simulink model "quadcopter"  (R2022b)
settings: Solver=VariableStepAuto  StartTime=0  StopTime=5  FixedStep=0.00000001  RelTol=1e-3  EnableMultiTasking=on
libraries: slpidlib x4, aerolibutil x2, shared6dof x1, aerolibanimutils x1, vrlib x1
settings Model: Creator=The MathWorks, Inc.  LastModifiedBy=aadri
settings SolverCC: AlgebraicLoopSolver=TrustRegion
settings DataIOCC: LimitDataPoints=on  SaveFormat=Array  SaveOutput=off  SignalLogging=off  DSMLogging=off  SaveTime=off  ReturnWorkspaceOutputs=off
settings OptimizationCC: BlockReduction=off  BufferReuse=off  LifeSpan=inf
settings DebuggingCC: AlgebraicLoopMsg=none  ParameterPrecisionLossMsg=none  AllowSymbolicDim=off  PregeneratedLibrarySubsystemCodeDiagnostic=none  SFUnexpectedBacktrackingDiag=warning  SFNoUnconditionalDefaultTransitionDiag=warning  SFExecutionAtInitializationDiag=none  SFMachineParentedDataDiag=warning  ArithmeticOperatorsInVariantConditions=warning
settings HardwareCC: ProdBitPerPointer=32  ProdBitPerSizeT=32  ProdBitPerPtrDiffT=32  ProdLargestAtomicFloat=None  ProdIntDivRoundTo=Undefined  ProdEndianess=Unspecified  ProdWordSize=32  ProdHWDeviceType=32-bit Generic
settings ModelReferenceCC: EnableRefExpFcnMdlSchedulingChecks=on  PropagateSignalLabelsOutOfModel=off
settings SFSimCC: SimUseLocalCustomCode=off  CustomCodeUndefinedFunction=UseInterfaceOnly
settings RTWCC: RTWUseLocalCustomCode=off  DLArmComputeVersion=19.05
settings CodeAppCC: StateflowObjectComments=on
settings GRTTargetCC: TargetLangStandard=C89/C90 (ANSI)
settings ConfigComp: CovMetricSettings=dw  CovSaveCumulativeToWorkspaceVar=on  CovSaveSingleToWorkspaceVar=on  CovExternalEMLEnable=off  CovSFcnEnable=off

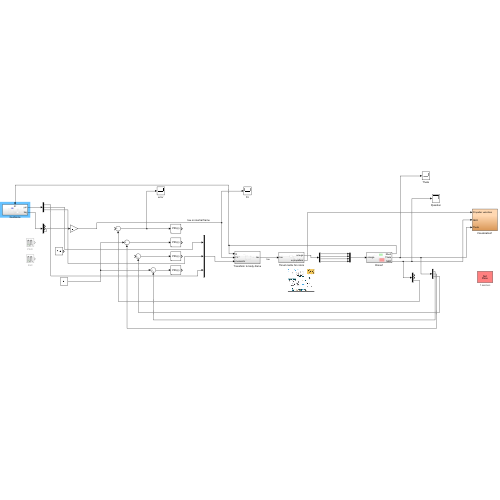
[thumbnail: Simulink's stored preview of the top-level diagram]
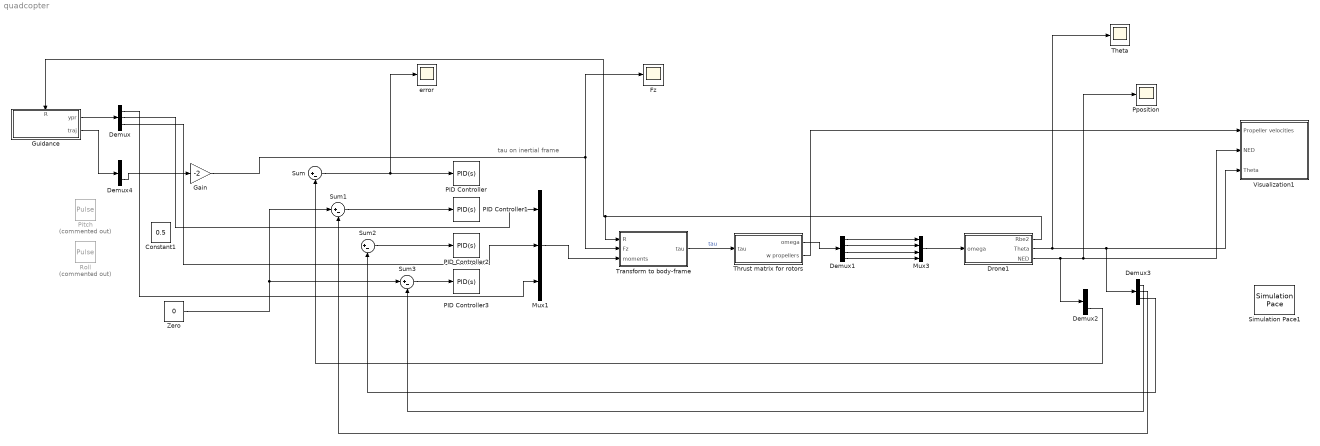
== system quadcopter ==
  note: tau on inertial frame
  Constant1 : Constant  Value=0.5
  Demux{,2..4} (4 alike) : Demux  Outputs=3
  Demux1 : Demux
  Drone1 : Subsystem
  Fz : Scope
  Gain : Gain  Gain=-2
  Guidance : Subsystem
      settings: PortSchema="{\"entries\":[{\"content\":{\"sides\":[{\"content\":{\"connectorIds\":[]},\"type\":\"ConnectorPlacement.EquallySpacedRectSide\",\"uuid\":\"71e90d44-93d9-4948-9515-e584c9c45b4d\"},{\"content\":{\"connectorIds\":[\"Out1\",\"Out2\"],\"side\":\"RIGHT\"},\"type\":\"ConnectorPlacement.EquallySpacedRectSide\",\"uuid\":\"b9ea6ff8-0025-4fb1-8de2-d026a39c77e0\"},{\"content\":{\"connectorIds\":[\"In1\"],\"side\":\"TOP\"},\"type\":\"ConnectorPlacement.EquallySpacedRectSide\",\"uuid\":\"2df58e0f-8a84-452f-95a8-5600226ef525\"}]},\"type\":\"ConnectorPlacement.EquallySpacedConnector\",\"uuid\":\"56107e1d-4b44-4050-8dfa-9220952eccff\"}],\"packageUris\":[\"http://schema.mathworks.com/mf0/Connector/R2020b\"],\"version\":\"1.0\"}"
  Mux1 : Mux  Inputs=3
  Mux3 : Mux
  PID Controller : slpidlib/PID Controller  Controller=PID  Form=Parallel  TimeDomain=Continuous-time  UseExternalTs=off  SampleTime=-1  IntegratorMethod=Forward Euler  FilterMethod=Forward Euler  ControllerParametersSource=internal  P=2  I=0  UseKiTs=off  D=0.5  N=100  UseFilter=on  TunerSelectOption=Transfer Function Based (PID Tuner App)  InitialConditionSource=internal  InitialConditionForIntegrator=0  InitialConditionForFilter=0  DifferentiatorICPrevScaledInput=0  ExternalReset=none  TrackingMode=off  Kt=1  LimitOutput=off  SatLimitsSource=internal  UpperSaturationLimit=5  LowerSaturationLimit=-5  LinearizeAsGain=on  AntiWindupMode=none  Kb=1  LimitIntegrator=off  UpperIntegratorSaturationLimit=inf  LowerIntegratorSaturationLimit=-inf  POutMin=[]  POutMax=[]  IOutMin=[]  IOutMax=[]  DOutMin=[]  DOutMax=[]  NOutMin=[]  NOutMax=[]  SumOutMin=[]  SumOutMax=[]  SaturationOutMin=[]  SaturationOutMax=[]  PParamMin=[]  PParamMax=[]  IParamMin=[]  IParamMax=[]  DParamMin=[]  DParamMax=[]  NParamMin=[]  NParamMax=[]  KbParamMin=[]  KbParamMax=[]  KtParamMin=[]  KtParamMax=[]  KbOutMin=[]  KbOutMax=[]  KtOutMin=[]  KtOutMax=[]  IntegratorOutMin=[]  IntegratorOutMax=[]  FilterOutMin=[]  FilterOutMax=[]  SumI1OutMin=[]  SumI1OutMax=[]  SumI2OutMin=[]  SumI2OutMax=[]  SumI3OutMin=[]  SumI3OutMax=[]  SumI4OutMin=[]  SumI4OutMax=[]  SumDOutMin=[]  SumDOutMax=[]  DifferentiatorOutMin=[]  DifferentiatorOutMax=[]  FilterDiffOutCoefMin=[]  FilterDiffOutCoefMax=[]  ReciprocalOutMin=[]  ReciprocalOutMax=[]  SumDenOutMin=[]  SumDenOutMax=[]  SumNumOutMin=[]  SumNumOutMax=[]  DivideOutMin=[]  DivideOutMax=[]  UdiffTsProdOutMin=[]  UdiffTsProdOutMax=[]  NTsProdOutMin=[]  NTsProdOutMax=[]  UintegralTsProdOutMin=[]  UintegralTsProdOutMax=[]  UngainTsProdOutMin=[]  UngainTsProdOutMax=[]  ClampingZeroOutDataTypeStr=Inherit: Inherit via back propagation  ClampingZeroOutMin=[]  ClampingZeroOutMax=[]  FilterDenConstantOutDataTypeStr=Inherit: Inherit via back propagation  FilterDenConstantOutMin=[]  FilterDenConstantOutMax=[]  PCopyOutDataTypeStr=Inherit: Inherit via back propagation  PCopyOutMin=[]  PCopyOutMax=[]  NCopyOutDataTypeStr=Inherit: Inherit via back propagation  NCopyOutMin=[]  NCopyOutMax=[]  IntegratorContinuousStateAttributes=''  IntegratorStateMustResolveToSignalObject=off  IntegratorRTWStateStorageClass=Auto  FilterContinuousStateAttributes=''  FilterStateMustResolveToSignalObject=off  FilterRTWStateStorageClass=Auto  ParallelPVariant=InternalParameters  IdealPVariant=Disabled  IVariant=InternalParameters  DVariant=InternalParameters  IntegratorVariant=Continuous  SatVariant=Disabled  AWVariant=Passthrough  PCopyVariant=Disabled  TRVariant=Disabled  FdbkBlocksVariant=Forward  IdealPFdbkVariant=Disabled  SatFdbkVariant=Disabled  DerivativeFilterVariant=ContFilter  NVariant=InternalParameters  NCopyVariant=Disabled  FilterICVariant=InternalICsFilter  IntegratorICVariant=InternalICs  ExternalResetVariant=Disabled  TRSumVariant=Passthrough  SumFdbkVariant=Disabled  SumVariant=Sum_PID  TsampFilterVariant=InternalTs  TsampNgainVariant=Passthrough  TsampIntegralVariant=Passthrough  ExternalSaturationOutDataTypeStr=Inherit: Same as second input
  PID Controller1 : slpidlib/PID Controller  Controller=PID  Form=Parallel  TimeDomain=Continuous-time  UseExternalTs=off  SampleTime=-1  IntegratorMethod=Forward Euler  FilterMethod=Forward Euler  ControllerParametersSource=internal  P=2  I=0  UseKiTs=off  D=0.5  N=100  UseFilter=on  TunerSelectOption=Transfer Function Based (PID Tuner App)  InitialConditionSource=internal  InitialConditionForIntegrator=0  InitialConditionForFilter=0  DifferentiatorICPrevScaledInput=0  ExternalReset=none  TrackingMode=off  Kt=1  LimitOutput=off  SatLimitsSource=internal  UpperSaturationLimit=inf  LowerSaturationLimit=-inf  LinearizeAsGain=on  AntiWindupMode=none  Kb=1  LimitIntegrator=off  UpperIntegratorSaturationLimit=inf  LowerIntegratorSaturationLimit=-inf  POutMin=[]  POutMax=[]  IOutMin=[]  IOutMax=[]  DOutMin=[]  DOutMax=[]  NOutMin=[]  NOutMax=[]  SumOutMin=[]  SumOutMax=[]  SaturationOutMin=[]  SaturationOutMax=[]  PParamMin=[]  PParamMax=[]  IParamMin=[]  IParamMax=[]  DParamMin=[]  DParamMax=[]  NParamMin=[]  NParamMax=[]  KbParamMin=[]  KbParamMax=[]  KtParamMin=[]  KtParamMax=[]  KbOutMin=[]  KbOutMax=[]  KtOutMin=[]  KtOutMax=[]  IntegratorOutMin=[]  IntegratorOutMax=[]  FilterOutMin=[]  FilterOutMax=[]  SumI1OutMin=[]  SumI1OutMax=[]  SumI2OutMin=[]  SumI2OutMax=[]  SumI3OutMin=[]  SumI3OutMax=[]  SumI4OutMin=[]  SumI4OutMax=[]  SumDOutMin=[]  SumDOutMax=[]  DifferentiatorOutMin=[]  DifferentiatorOutMax=[]  FilterDiffOutCoefMin=[]  FilterDiffOutCoefMax=[]  ReciprocalOutMin=[]  ReciprocalOutMax=[]  SumDenOutMin=[]  SumDenOutMax=[]  SumNumOutMin=[]  SumNumOutMax=[]  DivideOutMin=[]  DivideOutMax=[]  UdiffTsProdOutMin=[]  UdiffTsProdOutMax=[]  NTsProdOutMin=[]  NTsProdOutMax=[]  UintegralTsProdOutMin=[]  UintegralTsProdOutMax=[]  UngainTsProdOutMin=[]  UngainTsProdOutMax=[]  ClampingZeroOutDataTypeStr=Inherit: Inherit via back propagation  ClampingZeroOutMin=[]  ClampingZeroOutMax=[]  FilterDenConstantOutDataTypeStr=Inherit: Inherit via back propagation  FilterDenConstantOutMin=[]  FilterDenConstantOutMax=[]  PCopyOutDataTypeStr=Inherit: Inherit via back propagation  PCopyOutMin=[]  PCopyOutMax=[]  NCopyOutDataTypeStr=Inherit: Inherit via back propagation  NCopyOutMin=[]  NCopyOutMax=[]  IntegratorContinuousStateAttributes=''  IntegratorStateMustResolveToSignalObject=off  IntegratorRTWStateStorageClass=Auto  FilterContinuousStateAttributes=''  FilterStateMustResolveToSignalObject=off  FilterRTWStateStorageClass=Auto  ParallelPVariant=InternalParameters  IdealPVariant=Disabled  IVariant=InternalParameters  DVariant=InternalParameters  IntegratorVariant=Continuous  SatVariant=Disabled  AWVariant=Passthrough  PCopyVariant=Disabled  TRVariant=Disabled  FdbkBlocksVariant=Forward  IdealPFdbkVariant=Disabled  SatFdbkVariant=Disabled  DerivativeFilterVariant=ContFilter  NVariant=InternalParameters  NCopyVariant=Disabled  FilterICVariant=InternalICsFilter  IntegratorICVariant=InternalICs  ExternalResetVariant=Disabled  TRSumVariant=Passthrough  SumFdbkVariant=Disabled  SumVariant=Sum_PID  TsampFilterVariant=InternalTs  TsampNgainVariant=Passthrough  TsampIntegralVariant=Passthrough  ExternalSaturationOutDataTypeStr=Inherit: Same as second input
  PID Controller2 : slpidlib/PID Controller  Controller=PID  Form=Parallel  TimeDomain=Continuous-time  UseExternalTs=off  SampleTime=-1  IntegratorMethod=Forward Euler  FilterMethod=Forward Euler  ControllerParametersSource=internal  P=4  I=0  UseKiTs=off  D=2  N=100  UseFilter=on  TunerSelectOption=Transfer Function Based (PID Tuner App)  InitialConditionSource=internal  InitialConditionForIntegrator=0  InitialConditionForFilter=0  DifferentiatorICPrevScaledInput=0  ExternalReset=none  TrackingMode=off  Kt=1  LimitOutput=off  SatLimitsSource=internal  UpperSaturationLimit=inf  LowerSaturationLimit=-inf  LinearizeAsGain=on  AntiWindupMode=none  Kb=1  LimitIntegrator=off  UpperIntegratorSaturationLimit=inf  LowerIntegratorSaturationLimit=-inf  POutMin=[]  POutMax=[]  IOutMin=[]  IOutMax=[]  DOutMin=[]  DOutMax=[]  NOutMin=[]  NOutMax=[]  SumOutMin=[]  SumOutMax=[]  SaturationOutMin=[]  SaturationOutMax=[]  PParamMin=[]  PParamMax=[]  IParamMin=[]  IParamMax=[]  DParamMin=[]  DParamMax=[]  NParamMin=[]  NParamMax=[]  KbParamMin=[]  KbParamMax=[]  KtParamMin=[]  KtParamMax=[]  KbOutMin=[]  KbOutMax=[]  KtOutMin=[]  KtOutMax=[]  IntegratorOutMin=[]  IntegratorOutMax=[]  FilterOutMin=[]  FilterOutMax=[]  SumI1OutMin=[]  SumI1OutMax=[]  SumI2OutMin=[]  SumI2OutMax=[]  SumI3OutMin=[]  SumI3OutMax=[]  SumI4OutMin=[]  SumI4OutMax=[]  SumDOutMin=[]  SumDOutMax=[]  DifferentiatorOutMin=[]  DifferentiatorOutMax=[]  FilterDiffOutCoefMin=[]  FilterDiffOutCoefMax=[]  ReciprocalOutMin=[]  ReciprocalOutMax=[]  SumDenOutMin=[]  SumDenOutMax=[]  SumNumOutMin=[]  SumNumOutMax=[]  DivideOutMin=[]  DivideOutMax=[]  UdiffTsProdOutMin=[]  UdiffTsProdOutMax=[]  NTsProdOutMin=[]  NTsProdOutMax=[]  UintegralTsProdOutMin=[]  UintegralTsProdOutMax=[]  UngainTsProdOutMin=[]  UngainTsProdOutMax=[]  ClampingZeroOutDataTypeStr=Inherit: Inherit via back propagation  ClampingZeroOutMin=[]  ClampingZeroOutMax=[]  FilterDenConstantOutDataTypeStr=Inherit: Inherit via back propagation  FilterDenConstantOutMin=[]  FilterDenConstantOutMax=[]  PCopyOutDataTypeStr=Inherit: Inherit via back propagation  PCopyOutMin=[]  PCopyOutMax=[]  NCopyOutDataTypeStr=Inherit: Inherit via back propagation  NCopyOutMin=[]  NCopyOutMax=[]  IntegratorContinuousStateAttributes=''  IntegratorStateMustResolveToSignalObject=off  IntegratorRTWStateStorageClass=Auto  FilterContinuousStateAttributes=''  FilterStateMustResolveToSignalObject=off  FilterRTWStateStorageClass=Auto  ParallelPVariant=InternalParameters  IdealPVariant=Disabled  IVariant=InternalParameters  DVariant=InternalParameters  IntegratorVariant=Continuous  SatVariant=Disabled  AWVariant=Passthrough  PCopyVariant=Disabled  TRVariant=Disabled  FdbkBlocksVariant=Forward  IdealPFdbkVariant=Disabled  SatFdbkVariant=Disabled  DerivativeFilterVariant=ContFilter  NVariant=InternalParameters  NCopyVariant=Disabled  FilterICVariant=InternalICsFilter  IntegratorICVariant=InternalICs  ExternalResetVariant=Disabled  TRSumVariant=Passthrough  SumFdbkVariant=Disabled  SumVariant=Sum_PID  TsampFilterVariant=InternalTs  TsampNgainVariant=Passthrough  TsampIntegralVariant=Passthrough  ExternalSaturationOutDataTypeStr=Inherit: Same as second input
  PID Controller3 : slpidlib/PID Controller  Controller=PID  Form=Parallel  TimeDomain=Continuous-time  UseExternalTs=off  SampleTime=-1  IntegratorMethod=Forward Euler  FilterMethod=Forward Euler  ControllerParametersSource=internal  P=1  I=1  UseKiTs=off  D=0  N=100  UseFilter=on  TunerSelectOption=Transfer Function Based (PID Tuner App)  InitialConditionSource=internal  InitialConditionForIntegrator=0  InitialConditionForFilter=0  DifferentiatorICPrevScaledInput=0  ExternalReset=none  TrackingMode=off  Kt=1  LimitOutput=off  SatLimitsSource=internal  UpperSaturationLimit=inf  LowerSaturationLimit=-inf  LinearizeAsGain=on  AntiWindupMode=none  Kb=1  LimitIntegrator=off  UpperIntegratorSaturationLimit=inf  LowerIntegratorSaturationLimit=-inf  POutMin=[]  POutMax=[]  IOutMin=[]  IOutMax=[]  DOutMin=[]  DOutMax=[]  NOutMin=[]  NOutMax=[]  SumOutMin=[]  SumOutMax=[]  SaturationOutMin=[]  SaturationOutMax=[]  PParamMin=[]  PParamMax=[]  IParamMin=[]  IParamMax=[]  DParamMin=[]  DParamMax=[]  NParamMin=[]  NParamMax=[]  KbParamMin=[]  KbParamMax=[]  KtParamMin=[]  KtParamMax=[]  KbOutMin=[]  KbOutMax=[]  KtOutMin=[]  KtOutMax=[]  IntegratorOutMin=[]  IntegratorOutMax=[]  FilterOutMin=[]  FilterOutMax=[]  SumI1OutMin=[]  SumI1OutMax=[]  SumI2OutMin=[]  SumI2OutMax=[]  SumI3OutMin=[]  SumI3OutMax=[]  SumI4OutMin=[]  SumI4OutMax=[]  SumDOutMin=[]  SumDOutMax=[]  DifferentiatorOutMin=[]  DifferentiatorOutMax=[]  FilterDiffOutCoefMin=[]  FilterDiffOutCoefMax=[]  ReciprocalOutMin=[]  ReciprocalOutMax=[]  SumDenOutMin=[]  SumDenOutMax=[]  SumNumOutMin=[]  SumNumOutMax=[]  DivideOutMin=[]  DivideOutMax=[]  UdiffTsProdOutMin=[]  UdiffTsProdOutMax=[]  NTsProdOutMin=[]  NTsProdOutMax=[]  UintegralTsProdOutMin=[]  UintegralTsProdOutMax=[]  UngainTsProdOutMin=[]  UngainTsProdOutMax=[]  ClampingZeroOutDataTypeStr=Inherit: Inherit via back propagation  ClampingZeroOutMin=[]  ClampingZeroOutMax=[]  FilterDenConstantOutDataTypeStr=Inherit: Inherit via back propagation  FilterDenConstantOutMin=[]  FilterDenConstantOutMax=[]  PCopyOutDataTypeStr=Inherit: Inherit via back propagation  PCopyOutMin=[]  PCopyOutMax=[]  NCopyOutDataTypeStr=Inherit: Inherit via back propagation  NCopyOutMin=[]  NCopyOutMax=[]  IntegratorContinuousStateAttributes=''  IntegratorStateMustResolveToSignalObject=off  IntegratorRTWStateStorageClass=Auto  FilterContinuousStateAttributes=''  FilterStateMustResolveToSignalObject=off  FilterRTWStateStorageClass=Auto  ParallelPVariant=InternalParameters  IdealPVariant=Disabled  IVariant=InternalParameters  DVariant=InternalParameters  IntegratorVariant=Continuous  SatVariant=Disabled  AWVariant=Passthrough  PCopyVariant=Disabled  TRVariant=Disabled  FdbkBlocksVariant=Forward  IdealPFdbkVariant=Disabled  SatFdbkVariant=Disabled  DerivativeFilterVariant=ContFilter  NVariant=InternalParameters  NCopyVariant=Disabled  FilterICVariant=InternalICsFilter  IntegratorICVariant=InternalICs  ExternalResetVariant=Disabled  TRSumVariant=Passthrough  SumFdbkVariant=Disabled  SumVariant=Sum_PID  TsampFilterVariant=InternalTs  TsampNgainVariant=Passthrough  TsampIntegralVariant=Passthrough  ExternalSaturationOutDataTypeStr=Inherit: Same as second input
  Pitch : DiscretePulseGenerator  Commented=on  PulseType=Time based  Amplitude=-0.15  Period=1  PulseWidth=5  PhaseDelay=0.6
  Pposition : Scope
  Roll : DiscretePulseGenerator  Commented=on  PulseType=Time based  Amplitude=0.1  Period=10  PulseWidth=5  PhaseDelay=4
  Simulation Pace1 : aerolibanimutils/Simulation Pace  SimulationPace=1  SleepMode=MATLAB Thread  OutputPaceError=off  SampleTime=0.005
      settings: AttributesFormatString=%<SimulationPace> sec/sec
  Sum{,1..3} (4 alike) : Sum  Inputs=|+-
  Theta : Scope
  Thrust matrix for rotors : Subsystem
  Transform to body-frame : Subsystem
  Visualization1 : Subsystem
  Zero : Constant  Value=0  OutDataTypeStr=Inherit: Inherit via back propagation
  error : Scope
  wires:
  Sum/1 -> error/1, PID Controller/1
  Sum3/1 -> PID Controller3/1
  Drone1/3(NED) -> Demux2/1, Pposition/1, Visualization1/2(NED)
  Demux1/4 -> Mux3/4
  Demux1/3 -> Mux3/3
  Demux1/1 -> Mux3/1
  Mux3/1 -> Drone1/1(omega)
  Transform to body-frame/1(tau) -> Thrust matrix for rotors/1(tau)  "tau"
  Demux1/2 -> Mux3/2
  Sum2/1 -> PID Controller2/1
  Demux2/3 -> Sum/2
  Thrust matrix for rotors/1(omega) -> Demux1/1
  Sum1/1 -> PID Controller1/1
  Drone1/2(Theta) -> Theta/1, Demux3/1, Visualization1/3(Theta)
  Demux3/1 -> Sum3/2
  Demux3/2 -> Sum1/2
  Demux3/3 -> Sum2/2
  Drone1/1(Rbe2) -> Guidance/1(R), Transform to body-frame/1(R)
  Mux1/1 -> Transform to body-frame/3(moments)
  Thrust matrix for rotors/2(w propellers) -> Visualization1/1(Propeller velocities)
  Guidance/1(ypr) -> Demux/1
  Guidance/2(traj) -> Demux4/1
  Demux4/3 -> Gain/1
  Demux/3 -> Mux1/2
  Demux/1 -> Mux1/3
  Demux/2 -> Mux1/1
  Zero/1 -> Sum3/1, Sum1/1
  Gain/1 -> Fz/1, Transform to body-frame/2(Fz)

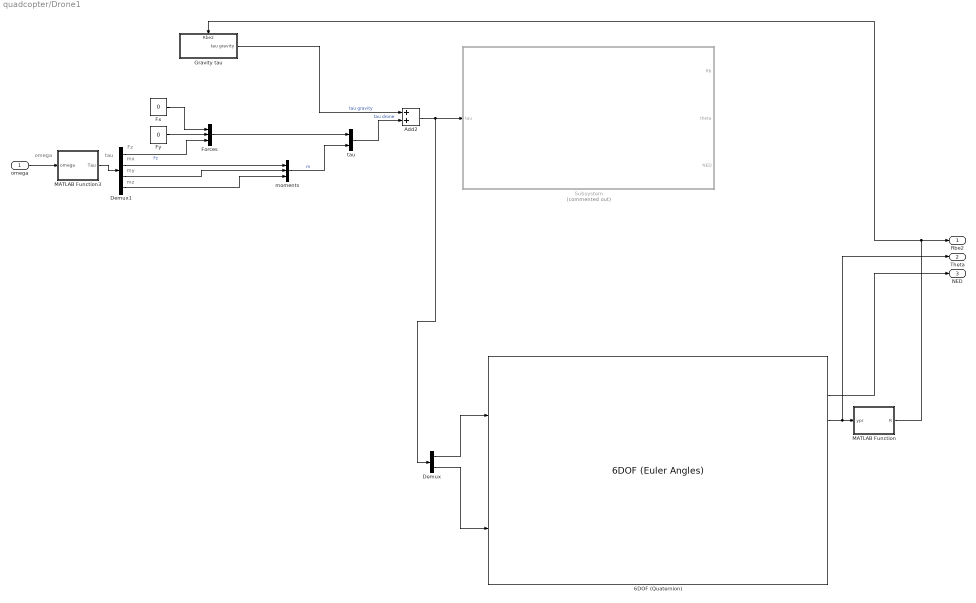
== system quadcopter/Drone1 ==
  note: mx
  note: Fz
  note: omega
  note: tau
  note: my
  note: mz
  omega : Inport
  6DOF (Quaternion) : shared6dof/6DOF (Euler Angles)  units=Metric (MKS)  mtype=Fixed  rep=Euler Angles  xme_0=init.posNED  Vm_0=init.vb  eul_0=init.euler  pm_0=init.angRates  mass_0=Vehicle.Airframe.mass  mass_e=0.5  mass_f=2.0  inertia=Vehicle.Airframe.inertia  inertia_e=eye(3)  inertia_f=2*eye(3)  k_quat=Vehicle.SixDOF.quatGain  vre_flag=on  abi_flag=on  aMode=aMode  xme_statename=''  Vm_statename=''  eul_statename=''  quat_statename=''  pm_statename=''  mass_statename=''
  Add2 : Sum
  Demux : Demux  Outputs=2
  Demux1 : Demux
  Forces : Mux  Inputs=3
  Fx : Constant  Value=0
  Fy : Constant  Value=0
  Gravity tau : Subsystem
      settings: PortSchema="{\"entries\":[{\"content\":{\"sides\":[{\"content\":{\"connectorIds\":[]},\"type\":\"ConnectorPlacement.EquallySpacedRectSide\",\"uuid\":\"34476b71-9b24-4b80-93b9-db525faab568\"},{\"content\":{\"connectorIds\":[\"Out1\"],\"side\":\"RIGHT\"},\"type\":\"ConnectorPlacement.EquallySpacedRectSide\",\"uuid\":\"f9e648e7-9cce-40ff-8639-1a2f2272512c\"},{\"content\":{\"connectorIds\":[\"In1\"],\"side\":\"TOP\"},\"type\":\"ConnectorPlacement.EquallySpacedRectSide\",\"uuid\":\"706437ea-9124-4f20-99e4-286431f5f4e3\"}]},\"type\":\"ConnectorPlacement.EquallySpacedConnector\",\"uuid\":\"20ce1a05-06ad-40f2-848e-d017002622b7\"}],\"packageUris\":[\"http://schema.mathworks.com/mf0/Connector/R2020b\"],\"version\":\"1.0\"}"
  MATLAB Function : MATLAB Function  TreatAsAtomicUnit=on
  MATLAB Function3 : MATLAB Function  TreatAsAtomicUnit=on
  Subsystem : Subsystem  Commented=on
  moments : Mux  Inputs=3
  tau : Mux  Inputs=2
  Rbe2 : Outport
  Theta : Outport  Port=2
  NED : Outport  Port=3
  wires:
  Demux1/2 -> moments/1
  Demux1/3 -> moments/2
  Demux1/4 -> moments/3
  MATLAB Function3/1(Tau) -> Demux1/1
  omega/1 -> MATLAB Function3/1(omega)
  Demux1/1 -> Forces/3  "Fz"
  Fy/1 -> Forces/2
  Fx/1 -> Forces/1
  Forces/1 -> tau/1
  moments/1 -> tau/2  "m"
  Gravity tau/1(tau gravity) -> Add2/1  "tau gravity"
  tau/1 -> Add2/2  "tau drone"
  Add2/1 -> Demux/1, Subsystem/1(tau)
  Demux/1 -> 6DOF (Quaternion)/1
  Demux/2 -> 6DOF (Quaternion)/2
  6DOF (Quaternion)/3 -> Theta/1, MATLAB Function/1(ypr)
  MATLAB Function/1(R) -> Gravity tau/1(Rbe2), Rbe2/1
  6DOF (Quaternion)/2 -> NED/1

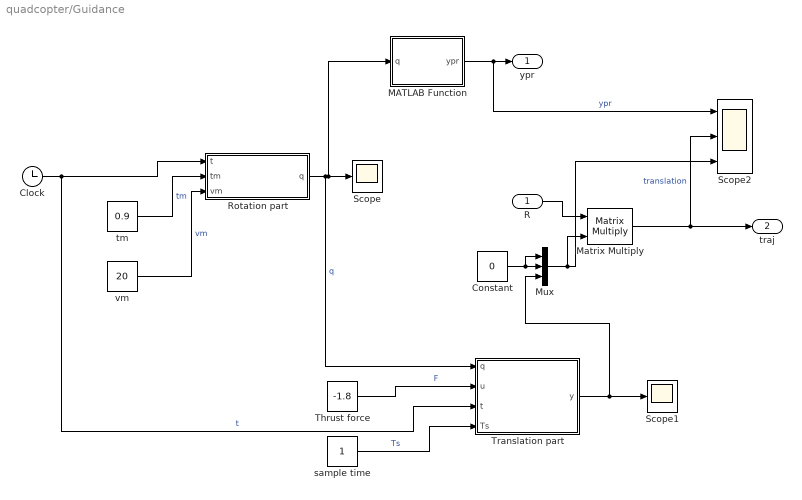
== system quadcopter/Guidance ==
  R : Inport
  Clock : Clock
  Constant : Constant  Value=0
  MATLAB Function : MATLAB Function  TreatAsAtomicUnit=on
  Matrix Multiply : Product  Multiplication=Matrix(*)
  Mux : Mux  Inputs=3
  Rotation part : Subsystem
  Scope : Scope
  Scope1 : Scope
  Scope2 : Scope  NumInputPorts=3
  Thrust force : Constant  Value=-1.8
  Translation part : Subsystem
  sample time : Constant
  tm : Constant  Value=0.9
  vm : Constant  Value=20
  ypr : Outport
  traj : Outport  Port=2
  wires:
  Clock/1 -> Translation part/3(t), Rotation part/1(t)  "t"
  tm/1 -> Rotation part/2(tm)  "tm"
  vm/1 -> Rotation part/3(vm)  "vm"
  Rotation part/1(q) -> Translation part/1(q), MATLAB Function/1(q), Scope/1  "q"
  Thrust force/1 -> Translation part/2(u)  "F"
  sample time/1 -> Translation part/4(Ts)  "Ts"
  Translation part/1(y) -> Mux/3, Scope1/1
  MATLAB Function/1(ypr) -> Scope2/1, ypr/1  "ypr"
  R/1 -> Matrix Multiply/1
  Constant/1 -> Mux/2, Mux/1
  Matrix Multiply/1 -> Scope2/2, traj/1  "translation"
  Mux/1 -> Scope2/3, Matrix Multiply/2

== system quadcopter/Thrust matrix for rotors ==
  note: omega
  note: tau
  tau : Inport
  MATLAB Function : MATLAB Function  TreatAsAtomicUnit=on
  MATLAB Function1 : MATLAB Function  TreatAsAtomicUnit=on
  omega : Outport
  w propellers : Outport  Port=2
  wires:
  tau/1 -> MATLAB Function/1(tau)
  MATLAB Function/1(omega) -> MATLAB Function1/1(omega), omega/1
  MATLAB Function1/1(w) -> w propellers/1

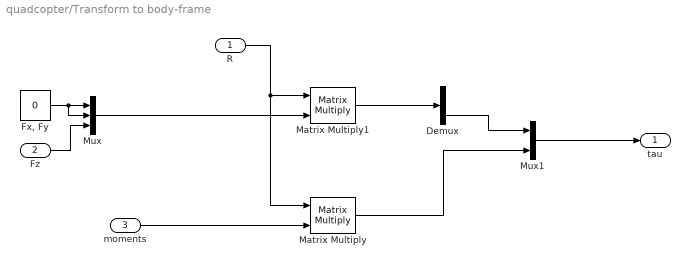
== system quadcopter/Transform to body-frame ==
  R : Inport
  Fz : Inport  Port=2
  moments : Inport  Port=3
  Demux : Demux  Outputs=3
  "Fx, Fy" : Constant  Value=0
  Matrix Multiply : Product  Multiplication=Matrix(*)
  Matrix Multiply1 : Product  Multiplication=Matrix(*)
  Mux : Mux  Inputs=3
  Mux1 : Mux  Inputs=2
  tau : Outport
  wires:
  "Fx, Fy"/1 -> Mux/2, Mux/1
  Fz/1 -> Mux/3
  R/1 -> Matrix Multiply/1, Matrix Multiply1/1
  Mux/1 -> Matrix Multiply1/2
  moments/1 -> Matrix Multiply/2
  Matrix Multiply1/1 -> Demux/1
  Mux1/1 -> tau/1
  Demux/3 -> Mux1/1
  Matrix Multiply/1 -> Mux1/2

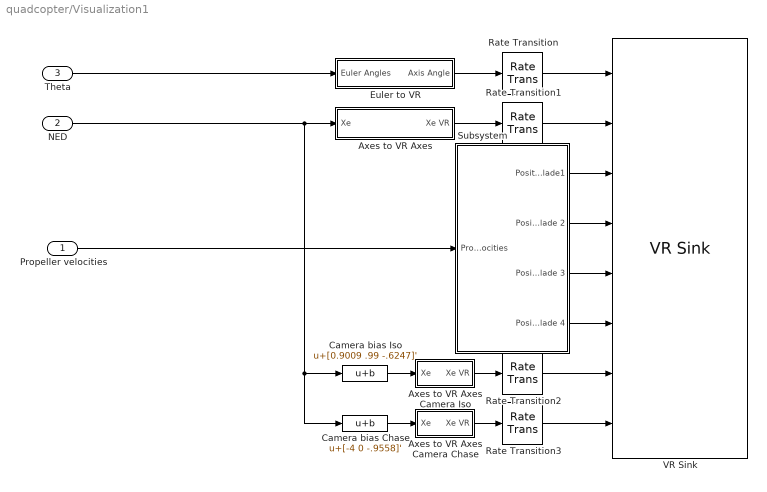
== system quadcopter/Visualization1 ==
  Propeller velocities : Inport
  NED : Inport  Port=2
  Theta : Inport  Port=3
  Axes to VR Axes : Subsystem
  Axes to VR Axes Camera Chase : Subsystem
  Axes to VR Axes Camera Iso : Subsystem
  Camera bias Chase : Bias  Bias=[-4 0 -.9558]'  SaturateOnIntegerOverflow=off
  Camera bias Iso : Bias  Bias=[0.9009 .99 -.6247]'  SaturateOnIntegerOverflow=off
  Euler to VR : Subsystem
  Rate Transition{,1..3} (4 alike) : RateTransition
  Subsystem : Subsystem
  VR Sink : vrlib/VR Sink  InstantiateOnLoad=on  SampleTime=12*0.005  ViewEnable=on  RemoteChange=off  RemoteView=off  FieldsWritten=QuadBody.rotation.4.1.1.double#QuadBody.translation.3.1.1.double#Blade1.rotation.4.1.1.double#Blade3.rotation.4.1.1.double#Blade2.rotation.4.1.1.double#Blade4.rotation.4.1.1.double#IsoNoRotation.position.3.1.1.double#OnQuadNoRotation.position.3.1.1.double  WorldFileName=Quadcopter_VR.wrl  AutoView=on  VideoDimensions=[]  AllowVariableSize=off  FigureProperties="{'Position', 'Name', 'Viewpoint', 'CameraBound', 'CameraDirection', 'CameraPosition', 'CameraUpVector', 'ZoomFactor', 'Antialiasing', 'Headlight', 'Lighting', 'NavPanel', 'Sound', 'StatusBar', 'Stereo3D', 'Stereo3DCameraOffset', 'Stereo3DHIT', 'ToolBar', 'Textures', 'Transparency', 'Triad', 'Wireframe', 'NavZones', 'NavMode', 'NavSpeed', 'CaptureFileFormat', 'CaptureFileName', 'Record2DCompressMethod', 'Record2DCompressQuality', 'Record2D', 'Record2DFileName', 'Record2DFPS'; [1.9871428571428569e+02   4.2642857142857133e+02   5.7600000000000000e+02   3.5000000000000006e+02], '', 'Isometric', 'on', [0.0000000000000000e+00   0.0000000000000000e+00  -1.0000000000000000e+00], [0.0000000000000000e+00   0.0000000000000000e+00   3.0000000000000000e+00], [0.0000000000000000e+00   1.0000000000000000e+00   0.0000000000000000e+00], [1.0000000000000000e+00], 'on', 'on', 'on', 'halfbar', 'on', 'on', 'off', [1.0000000149011612e-01], [0.0000000000000000e+00], 'on', 'on', 'on', 'none', 'off', 'off', 'fly', 'normal', 'tif', '%f_anim_%n.tif', 'auto', [7.5000000000000000e+01], 'off', '%f_anim_%n.avi', 'auto'}"
  wires:
  Propeller velocities/1 -> Subsystem/1(Propeller velocities)
  Euler to VR/1(Axis Angle) -> Rate Transition/1
  Axes to VR Axes/1(Xe VR) -> Rate Transition1/1
  Camera bias Iso/1 -> Axes to VR Axes Camera Iso/1(Xe)
  Camera bias Chase/1 -> Axes to VR Axes Camera Chase/1(Xe)
  Axes to VR Axes Camera Chase/1(Xe VR) -> Rate Transition3/1
  NED/1 -> Camera bias Chase/1, Camera bias Iso/1, Axes to VR Axes/1(Xe)
  Axes to VR Axes Camera Iso/1(Xe VR) -> Rate Transition2/1
  Theta/1 -> Euler to VR/1(Euler Angles)
  Rate Transition/1 -> VR Sink/1
  Rate Transition1/1 -> VR Sink/2
  Subsystem/1(Position Blade1) -> VR Sink/3
  Subsystem/2(Position Blade 2) -> VR Sink/4
  Subsystem/3(Position Blade 3) -> VR Sink/5
  Subsystem/4(Position Blade 4) -> VR Sink/6
  Rate Transition2/1 -> VR Sink/7
  Rate Transition3/1 -> VR Sink/8

== system quadcopter/Drone1/Gravity tau ==
  Rbe2 : Inport
  Constant1 : Constant  Value=[0;0;0.28*9.81]
  Constant2 : Constant  Value=[0;0;0]
  Matrix Multiply : Product  Multiplication=Matrix(*)
  Mux : Mux  Inputs=2
  tau gravity : Outport
  wires:
  Rbe2/1 -> Matrix Multiply/1
  Matrix Multiply/1 -> Mux/1  "tau gravity"
  Mux/1 -> tau gravity/1
  Constant1/1 -> Matrix Multiply/2
  Constant2/1 -> Mux/2

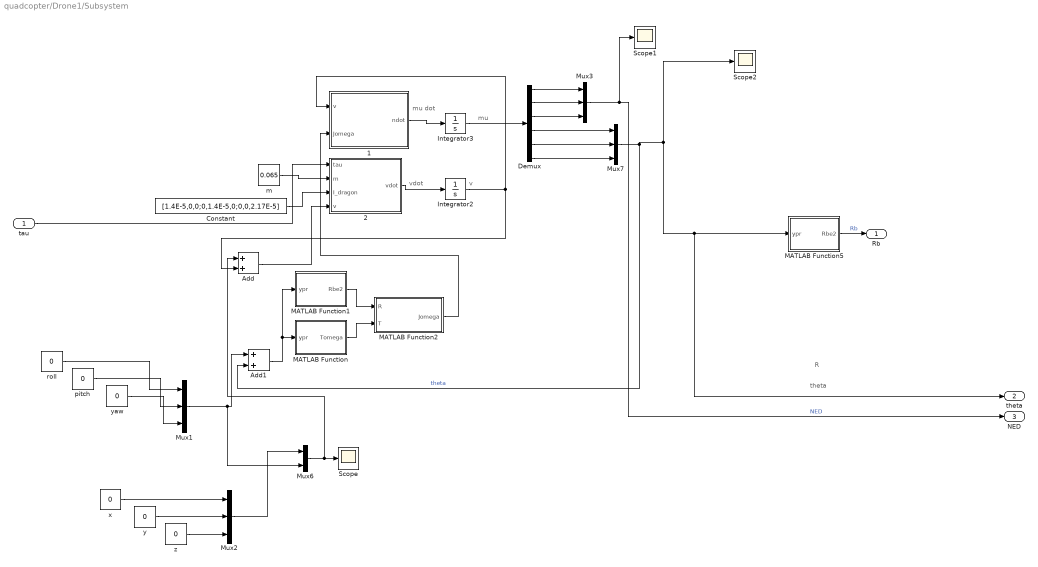
== system quadcopter/Drone1/Subsystem ==
  note: theta
  note: R
  note: mu dot
  note: mu
  note: v
  note: vdot
  tau : Inport
  1 : MATLAB Function  TreatAsAtomicUnit=on
  2 : MATLAB Function  TreatAsAtomicUnit=on
  Add : Sum
  Add1 : Sum
  Constant : Constant  Value=[1.4E-5,0,0;0,1.4E-5,0;0,0,2.17E-5]
  Demux : Demux  Outputs=6
  Integrator2 : Integrator
  Integrator3 : Integrator
  MATLAB Function : MATLAB Function  TreatAsAtomicUnit=on
  MATLAB Function1 : MATLAB Function  TreatAsAtomicUnit=on
  MATLAB Function2 : MATLAB Function  TreatAsAtomicUnit=on
  MATLAB Function5 : MATLAB Function  TreatAsAtomicUnit=on
  Mux{1..3,7} (4 alike) : Mux  Inputs=3
  Mux6 : Mux  Inputs=2
  Scope : Scope
  Scope1 : Scope
  Scope2 : Scope
  m : Constant  Value=0.065
  pitch : Constant  Value=0
  roll : Constant  Value=0
  x : Constant  Value=0
  y : Constant  Value=0
  yaw : Constant  Value=0
  z : Constant  Value=0
  Rb : Outport
  theta : Outport  Port=2
  NED : Outport  Port=3
  wires:
  Integrator3/1 -> Demux/1
  Demux/5 -> Mux7/2
  m/1 -> 2/2(m)
  pitch/1 -> Mux1/2
  Mux1/1 -> Mux6/2, Add1/1
  yaw/1 -> Mux1/3
  Demux/6 -> Mux7/3
  Mux6/1 -> Add/1, Scope/1
  tau/1 -> 2/1(tau)
  Mux7/1 -> Add1/2, theta/1, MATLAB Function5/1(ypr), Scope2/1  "theta"
  Integrator2/1 -> 1/1(v), Add/2
  Mux3/1 -> NED/1, Scope1/1  "NED"
  MATLAB Function/1(Tomega) -> MATLAB Function2/2(T)
  2/1(vdot) -> Integrator2/1
  Add/1 -> 2/4(v)
  Demux/1 -> Mux3/1
  1/1(ndot) -> Integrator3/1
  Add1/1 -> MATLAB Function/1(ypr), MATLAB Function1/1(ypr)
  MATLAB Function2/1(Jomega) -> 1/2(Jomega)
  z/1 -> Mux2/3
  MATLAB Function1/1(Rbe2) -> MATLAB Function2/1(R)
  x/1 -> Mux2/1
  Demux/4 -> Mux7/1
  roll/1 -> Mux1/1
  Constant/1 -> 2/3(I_dragon)
  Mux2/1 -> Mux6/1
  Demux/3 -> Mux3/3
  Demux/2 -> Mux3/2
  y/1 -> Mux2/2
  MATLAB Function5/1(Rbe2) -> Rb/1  "Rb"

== system quadcopter/Guidance/Rotation part ==
  t : Inport
  tm : Inport  Port=2
  vm : Inport  Port=3
  MATLAB Function : MATLAB Function  TreatAsAtomicUnit=on
  q : Outport
  wires:
  t/1 -> MATLAB Function/1(t)
  tm/1 -> MATLAB Function/2(tm)
  vm/1 -> MATLAB Function/3(vm)
  MATLAB Function/1(q) -> q/1

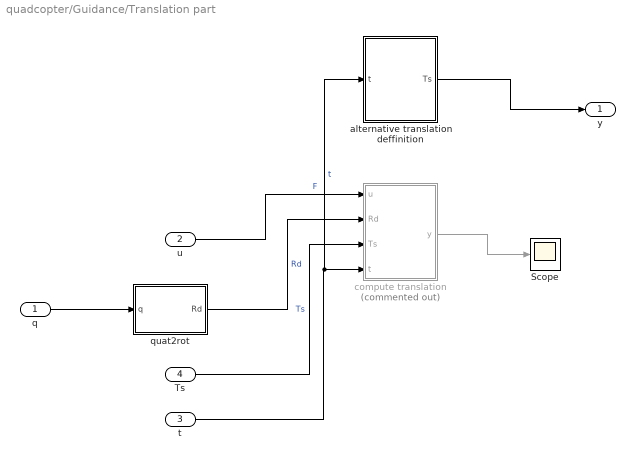
== system quadcopter/Guidance/Translation part ==
  q : Inport
  u : Inport  Port=2
  t : Inport  Port=3
  Ts : Inport  Port=4
  Scope : Scope
  alternative translation deffinition : MATLAB Function  TreatAsAtomicUnit=on
  compute translation : MATLAB Function  Commented=on  TreatAsAtomicUnit=on
  quat2rot : MATLAB Function  TreatAsAtomicUnit=on
  y : Outport
  wires:
  q/1 -> quat2rot/1(q)
  u/1 -> compute translation/1(u)  "F"
  quat2rot/1(Rd) -> compute translation/2(Rd)  "Rd"
  Ts/1 -> compute translation/3(Ts)  "Ts"
  t/1 -> alternative translation deffinition/1(t), compute translation/4(t)  "t"
  compute translation/1(y) -> Scope/1
  alternative translation deffinition/1(Ts) -> y/1

== system quadcopter/Visualization1/Axes to VR Axes ==
  Xe : Inport
  Demux : Demux  Outputs=3
      settings: DisplayOption=none
  Mux : Mux  Inputs=3
  rad-->deg1 : Gain  Gain=-1  SaturateOnIntegerOverflow=on  OutDataTypeStr=Inherit: Same as input  ParamDataTypeStr=Inherit: Same as input
  Xe VR : Outport  VectorParamsAs1DForOutWhenUnconnected=off
  wires:
  Xe/1 -> Demux/1
  Demux/1 -> Mux/1
  Demux/3 -> rad-->deg1/1
  Mux/1 -> Xe VR/1
  rad-->deg1/1 -> Mux/2
  Demux/2 -> Mux/3

== system quadcopter/Visualization1/Axes to VR Axes Camera Chase ==
  Xe : Inport
  Demux : Demux  Outputs=3
      settings: DisplayOption=none
  Mux : Mux  Inputs=3
  rad-->deg1 : Gain  Gain=-1  SaturateOnIntegerOverflow=on  OutDataTypeStr=Inherit: Same as input  ParamDataTypeStr=Inherit: Same as input
  Xe VR : Outport  VectorParamsAs1DForOutWhenUnconnected=off
  wires:
  Xe/1 -> Demux/1
  Demux/1 -> Mux/1
  Demux/3 -> rad-->deg1/1
  Mux/1 -> Xe VR/1
  rad-->deg1/1 -> Mux/2
  Demux/2 -> Mux/3

== system quadcopter/Visualization1/Axes to VR Axes Camera Iso ==
  Xe : Inport
  Demux : Demux  Outputs=3
      settings: DisplayOption=none
  Mux : Mux  Inputs=3
  rad-->deg1 : Gain  Gain=-1  SaturateOnIntegerOverflow=on  OutDataTypeStr=Inherit: Same as input  ParamDataTypeStr=Inherit: Same as input
  Xe VR : Outport  VectorParamsAs1DForOutWhenUnconnected=off
  wires:
  Demux/2 -> Mux/3
  rad-->deg1/1 -> Mux/2
  Mux/1 -> Xe VR/1
  Demux/3 -> rad-->deg1/1
  Demux/1 -> Mux/1
  Xe/1 -> Demux/1

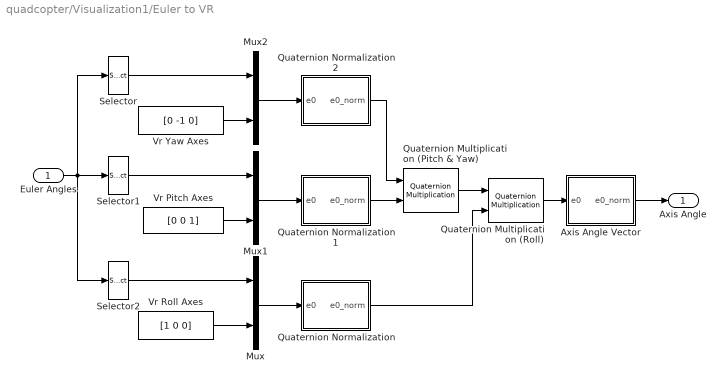
== system quadcopter/Visualization1/Euler to VR ==
  Euler Angles : Inport
  Axis Angle Vector : Subsystem
  Mux : Mux  Inputs=2
  Mux1 : Mux  Inputs=2
  Mux2 : Mux  Inputs=2
  Quaternion Multiplication (Pitch & Yaw) : aerolibutil/Quaternion Multiplication
  Quaternion Multiplication (Roll) : aerolibutil/Quaternion Multiplication
  Quaternion Normalization : Subsystem
  Quaternion Normalization1 : Subsystem
  Quaternion Normalization2 : Subsystem
  Selector : Selector  InputPortWidth=3  IndexOptions=Index vector (dialog)  Indices=[3]  OutputSizes=1
  Selector1 : Selector  InputPortWidth=3  IndexOptions=Index vector (dialog)  Indices=[2]  OutputSizes=1
  Selector2 : Selector  InputPortWidth=3  IndexOptions=Index vector (dialog)  Indices=[1]  OutputSizes=1
  Vr Pitch Axes : Constant  Value=[0 0 1]
  Vr Roll Axes : Constant  Value=[1 0 0]
  Vr Yaw Axes : Constant  Value=[0 -1 0]
  Axis Angle : Outport  VectorParamsAs1DForOutWhenUnconnected=off
  wires:
  Quaternion Multiplication (Roll)/1 -> Axis Angle Vector/1(e0)
  Axis Angle Vector/1(e0_norm) -> Axis Angle/1
  Quaternion Normalization/1(e0_norm) -> Quaternion Multiplication (Roll)/2
  Quaternion Normalization2/1(e0_norm) -> Quaternion Multiplication (Pitch & Yaw)/1
  Quaternion Normalization1/1(e0_norm) -> Quaternion Multiplication (Pitch & Yaw)/2
  Mux2/1 -> Quaternion Normalization2/1(e0)
  Mux1/1 -> Quaternion Normalization1/1(e0)
  Mux/1 -> Quaternion Normalization/1(e0)
  Selector/1 -> Mux2/1
  Vr Yaw Axes/1 -> Mux2/2
  Selector1/1 -> Mux1/1
  Vr Pitch Axes/1 -> Mux1/2
  Selector2/1 -> Mux/1
  Vr Roll Axes/1 -> Mux/2
  Euler Angles/1 -> Selector2/1, Selector1/1, Selector/1
  Quaternion Multiplication (Pitch & Yaw)/1 -> Quaternion Multiplication (Roll)/1

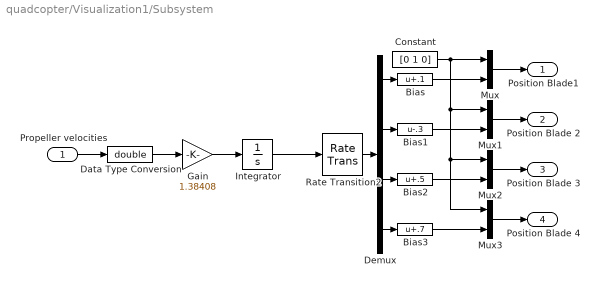
== system quadcopter/Visualization1/Subsystem ==
  Propeller velocities : Inport
  Bias : Bias  Bias=.1  SaturateOnIntegerOverflow=off
  Bias1 : Bias  Bias=-.3  SaturateOnIntegerOverflow=off
  Bias2 : Bias  Bias=.5  SaturateOnIntegerOverflow=off
  Bias3 : Bias  Bias=.7  SaturateOnIntegerOverflow=off
  Constant : Constant  Value=[0 1 0]
  Data Type Conversion : DataTypeConversion  OutDataTypeStr=double  SaturateOnIntegerOverflow=off  RndMeth=Floor
  Demux : Demux
  Gain : Gain  Gain=1.38408
  Integrator : Integrator  InitialCondition=[.1 ; .2 ;-.3 ;-.4]  WrapState=on  WrappedStateUpperValue=2*pi  WrappedStateLowerValue=-2*pi
  Mux{,1..3} (4 alike) : Mux  Inputs=2
  Rate Transition2 : RateTransition
  Position Blade1 : Outport  VectorParamsAs1DForOutWhenUnconnected=off
  Position Blade 2 : Outport  Port=2  VectorParamsAs1DForOutWhenUnconnected=off
  Position Blade 3 : Outport  Port=3  VectorParamsAs1DForOutWhenUnconnected=off
  Position Blade 4 : Outport  Port=4  VectorParamsAs1DForOutWhenUnconnected=off
  wires:
  Bias3/1 -> Mux3/2
  Mux3/1 -> Position Blade 4/1
  Bias1/1 -> Mux1/2
  Bias2/1 -> Mux2/2
  Demux/2 -> Bias1/1
  Constant/1 -> Mux3/1, Mux2/1, Mux1/1, Mux/1
  Mux1/1 -> Position Blade 2/1
  Mux2/1 -> Position Blade 3/1
  Integrator/1 -> Rate Transition2/1
  Mux/1 -> Position Blade1/1
  Demux/3 -> Bias2/1
  Bias/1 -> Mux/2
  Propeller velocities/1 -> Data Type Conversion/1
  Demux/4 -> Bias3/1
  Rate Transition2/1 -> Demux/1
  Demux/1 -> Bias/1
  Data Type Conversion/1 -> Gain/1
  Gain/1 -> Integrator/1

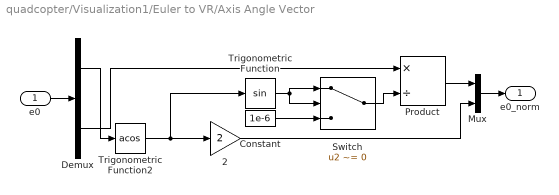
== system quadcopter/Visualization1/Euler to VR/Axis Angle Vector ==
  e0 : Inport
  2 : Gain  Gain=2  SaturateOnIntegerOverflow=on  OutDataTypeStr=Inherit: Same as input  ParamDataTypeStr=Inherit: Same as input
  Constant : Constant  Value=1e-6
  Demux : Demux  Outputs=[1 3 ]
      settings: DisplayOption=none
  Mux : Mux  Inputs=2
  Product : Product  Inputs=*/  InputSameDT=on  SaturateOnIntegerOverflow=on  OutDataTypeStr=Inherit: Same as first input
  Switch : Switch  Criteria=u2 ~= 0  SaturateOnIntegerOverflow=off  InputSameDT=off
  Trigonometric Function : Trigonometry
  Trigonometric Function2 : Trigonometry  Operator=acos
  e0_norm : Outport  VectorParamsAs1DForOutWhenUnconnected=off
  wires:
  Demux/1 -> Trigonometric Function2/1
  Demux/2 -> Product/1
  Mux/1 -> e0_norm/1
  Product/1 -> Mux/1
  2/1 -> Mux/2
  Trigonometric Function/1 -> Switch/1, Switch/2
  Trigonometric Function2/1 -> Trigonometric Function/1, 2/1
  e0/1 -> Demux/1
  Constant/1 -> Switch/3
  Switch/1 -> Product/2

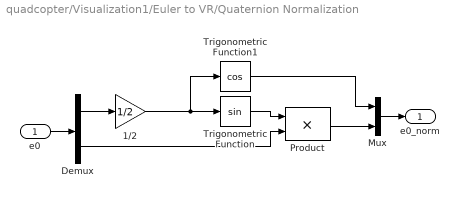
== system quadcopter/Visualization1/Euler to VR/Quaternion Normalization ==
  e0 : Inport
  1/2 : Gain  Gain=1/2  SaturateOnIntegerOverflow=on  OutDataTypeStr=Inherit: Same as input  ParamDataTypeStr=Inherit: Same as input
  Demux : Demux  Outputs=[1 3]
      settings: DisplayOption=none
  Mux : Mux  Inputs=2
  Product : Product  InputSameDT=on  SaturateOnIntegerOverflow=on  OutDataTypeStr=Inherit: Same as first input
  Trigonometric Function : Trigonometry
  Trigonometric Function1 : Trigonometry  Operator=cos
  e0_norm : Outport  VectorParamsAs1DForOutWhenUnconnected=off
  wires:
  Trigonometric Function1/1 -> Mux/1
  Demux/2 -> Product/2
  Demux/1 -> 1/2/1
  Mux/1 -> e0_norm/1
  Product/1 -> Mux/2
  Trigonometric Function/1 -> Product/1
  1/2/1 -> Trigonometric Function1/1, Trigonometric Function/1
  e0/1 -> Demux/1

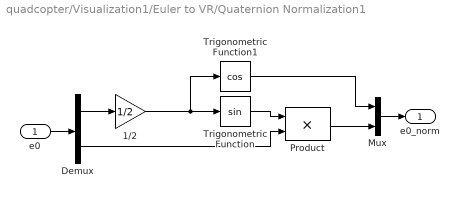
== system quadcopter/Visualization1/Euler to VR/Quaternion Normalization1 ==
  e0 : Inport
  1/2 : Gain  Gain=1/2  SaturateOnIntegerOverflow=on  OutDataTypeStr=Inherit: Same as input  ParamDataTypeStr=Inherit: Same as input
  Demux : Demux  Outputs=[1 3]
      settings: DisplayOption=none
  Mux : Mux  Inputs=2
  Product : Product  InputSameDT=on  SaturateOnIntegerOverflow=on  OutDataTypeStr=Inherit: Same as first input
  Trigonometric Function : Trigonometry
  Trigonometric Function1 : Trigonometry  Operator=cos
  e0_norm : Outport  VectorParamsAs1DForOutWhenUnconnected=off
  wires:
  e0/1 -> Demux/1
  1/2/1 -> Trigonometric Function/1, Trigonometric Function1/1
  Trigonometric Function/1 -> Product/1
  Product/1 -> Mux/2
  Mux/1 -> e0_norm/1
  Demux/1 -> 1/2/1
  Demux/2 -> Product/2
  Trigonometric Function1/1 -> Mux/1

== system quadcopter/Visualization1/Euler to VR/Quaternion Normalization2 ==
  e0 : Inport
  1/2 : Gain  Gain=1/2  SaturateOnIntegerOverflow=on  OutDataTypeStr=Inherit: Same as input  ParamDataTypeStr=Inherit: Same as input
  Demux : Demux  Outputs=[1 3]
      settings: DisplayOption=none
  Mux : Mux  Inputs=2
  Product : Product  InputSameDT=on  SaturateOnIntegerOverflow=on  OutDataTypeStr=Inherit: Same as first input
  Trigonometric Function : Trigonometry
  Trigonometric Function1 : Trigonometry  Operator=cos
  e0_norm : Outport  VectorParamsAs1DForOutWhenUnconnected=off
  wires:
  Trigonometric Function1/1 -> Mux/1
  Demux/2 -> Product/2
  Demux/1 -> 1/2/1
  Mux/1 -> e0_norm/1
  Product/1 -> Mux/2
  Trigonometric Function/1 -> Product/1
  1/2/1 -> Trigonometric Function1/1, Trigonometric Function/1
  e0/1 -> Demux/1

== matlab function quadcopter/Thrust matrix for rotors/MATLAB Function1 ==
  data: omega input; w output
function w = fcn(omega)

k = 2.88E-8;

w1 = omega(1)/k;
w2 = omega(2)/k;
w3 = omega(3)/k;
w4 = omega(4)/k;

w = [w1; w2; w3; w4];

== matlab function quadcopter/Drone1/MATLAB Function3 ==
  data: omega input; Tau output
function Tau = T(omega)

kt = 1;
km = 1;
lx = 4.2426;
ly = 4.2426;

l = 0.092;
b = 7.24E-10;
k = 2.88E-8;

% T = [-kt    -kt     -kt     -kt;
%     -ly*kt  ly*kt   ly*kt   -ly*kt;
%     lx*kt   -lx*kt  lx*kt   -lx*kt;
%     -km     -km     km      km];

T = [1    1     1     1;
    -l  -l   l   l;
    l   -l  -l   l;
    b/k     -b/k     b/k    -b/k];

Tau = T*omega;


end

== matlab function quadcopter/Drone1/Subsystem/MATLAB Function5 ==
  data: ypr input; Rbe2 output
function Rbe2 = RotMatrix2(ypr)
%UNTITLED Summary of this function goes here
%   Detailed explanation goes here


Rz = [cos(ypr(1)) -sin(ypr(1)) 0;
    sin(ypr(1)) cos(ypr(1)) 0;
    0   0   1];
Ry = [cos(ypr(2)) 0 sin(ypr(2));
    0   1   0;
    -sin(ypr(2)) 0 cos(ypr(2))];
Rx = [1     0   0;
    0 cos(ypr(3)) -sin(ypr(3));
    0 sin(ypr(3)) cos(ypr(3))];

Rbe2 = Rz*Ry*Rx;
end

== matlab function quadcopter/Thrust matrix for rotors/MATLAB Function ==
  data: tau input; omega output
function omega = MMAT(tau)

% kt = 1;
% km = 1;
% lx = 4.2426;
% ly = 4.2426;

l = 0.092;
b = 7.24E-10;
k = 2.88E-8;

% T = [-kt    -kt     -kt     -kt;
%     -ly*kt  ly*kt   ly*kt   -ly*kt;
%     lx*kt   -lx*kt  lx*kt   -lx*kt;
%     -km     -km     km      km];

T = [1    1     1     1;
    -l  -l   l   l;
    l   -l  -l   l;
    b/k     -b/k     b/k    -b/k];

omega = inv(T) * tau;

end

== matlab function quadcopter/Drone1/Subsystem/1 ==
  data: v input; ndot output; Jomega input
function ndot = ndotfunction(v, Jomega)

ndot = Jomega * v;

end

== matlab function quadcopter/Guidance/Rotation part/MATLAB Function ==
  data: t input; q output; tm input; vm input
function q = fcn(t, tm, vm)

q0d = (2/(1+exp(-vm*(t-tm/2))))-1;
q2d = sqrt(1-q0d^2);

q = [q0d, 0, q2d, 0];

end

== matlab function quadcopter/Guidance/Translation part/quat2rot ==
  data: q input; Rd output
function Rd = fcn(q)

quat = quaternion(q);

Rd = quat2rotm(quat)

end

== matlab function quadcopter/Guidance/Translation part/compute translation ==
  data: u input; y output; Rd input; Ts input; t input
function y = fcn(u, Rd, Ts, t)

persistent psi;
    if isempty(psi)
        psi = [-0.6;
                0;
                -0.5;
                0.45]-1.5;
    end
m = 0.028;
N = 432;

A = [1 Ts 0 0;
    0 1 0 0;
    0 0 1 Ts;
    0 0 0 1];

B = [Rd(1,3)*Ts^2/(2*m);
    Rd(1,3)*Ts/m;
    Rd(3,3)*Ts^2/(2*m);
    Rd(3,3)*Ts/m];

X_ = [-0.6;
    0;
    -0.5;
    0.45]-1.5;

C = [0, 0, 0, 1];


if t == 0
    psi_ = A*X_ + B*u;
    y = C * X_;
    psi = psi_;
% elseif t==N
%     f = zeros(2,2);
%     H = diag([1,0,1,0]);
%     A = [];
%     b = [];
%     Aeq = [1 Ts 0 0;
%     0 1 0 0;
%     0 0 1 Ts;
%     0 0 0 1];
%     beq = [-0.6;
%     0;
%     -0.5;
%     0.45]-1.5;
% 
%     lb = [];
%     ub = [];
% 
%     x0 = [0 0 0 0];
%     options = optimoptions('quadprog','Algorithm','active-set');
% 
%     x = quadprog(H,f,A,b, Aeq, beq, lb, ub, x0, options)
%     
%     y = [0, 0, 0 ,x]
%     % y = C * x;
else
    psi_ = A*psi + B*u;
    y = C * psi;
    psi = psi_
    
end

%psi = psi_;

== matlab function quadcopter/Guidance/Translation part/alternative translation deffinition ==
  data: t input; Ts output
function Ts = fcn(t)

% Define constants
g = 9.81; % Acceleration due to gravity
h = 1; % Height of flip
T = 1; % Total duration of flip
%t = linspace(0, T, 100); % Time vector

% Calculate desired velocity and acceleration profiles
v_desired = sqrt(2 * g * h) * sin(pi * t / T);
a_desired = (pi / T) * sqrt(2 * g * h) * cos(pi * t / T);

% Calculate desired position profile
x_desired = zeros(size(t));
y_desired = zeros(size(t));
z_desired = h - (g / 2) * (t.^2) + (h / pi) * (cos(pi * t / T) - 1);
Ts = sqrt(abs(z_desired)/(0.5*g))/(t+0.02);

== matlab function quadcopter/Drone1/Subsystem/2 ==
  data: tau input; m input; vdot output; I_dragon input; v input
function vdot = fcn(tau, m, I_dragon, v)

% if v == null
%     v = [1;1;1;1;1;1];
% end

%C
w = v(4:6,:);
wx = [0     -w(3,1)     w(2,1);
    w(3,1)    0         -w(1,1);
    -w(2,1)  w(1,1)         0];
Iw = I_dragon*w;
Iwx = [0     -Iw(3,1)     Iw(2,1);
    Iw(3,1)    0         -Iw(1,1);
    -Iw(2,1)  Iw(1,1)         0];

Cmat = [m*wx    zeros(3,3);
        zeros(3,3)  -Iwx];


%M
Mrb = [m*eye(3,3) zeros(3,3);
    zeros(3,3) I_dragon];

vdot = -Mrb^-1*Cmat*v + Mrb^-1*tau;


end

== matlab function quadcopter/Guidance/MATLAB Function ==
  data: q input; ypr output
function ypr = fcn(q)

p =  2*acos(q(1));

ypr = [0, p, 0];

== matlab function quadcopter/Drone1/MATLAB Function ==
  data: ypr input; R output
function R = fcn(ypr)

R = eul2rotm(ypr');

== matlab function quadcopter/Drone1/Subsystem/MATLAB Function ==
  data: ypr input; Tomega output
function Tomega = Tmat(ypr)



Tomega = [1         sin(ypr(3))*(sin(ypr(2))/cos(ypr(2)))       cos(ypr(3))*(sin(ypr(2))/cos(ypr(2)));
          0                     cos(ypr(2))                                 -sin(ypr(2));
          0                sin(ypr(3))/cos(ypr(2))                  cos(ypr(3))/cos(ypr(2))];

end

== matlab function quadcopter/Drone1/Subsystem/MATLAB Function1 ==
  data: ypr input; Rbe2 output
function Rbe2 = RotMatrix2(ypr)
%UNTITLED Summary of this function goes here
%   Detailed explanation goes here


Rz = [cos(ypr(1)) -sin(ypr(1)) 0;
    sin(ypr(1)) cos(ypr(1)) 0;
    0   0   1];
Ry = [cos(ypr(2)) 0 sin(ypr(2));
    0   1   0;
    -sin(ypr(2)) 0 cos(ypr(2))];
Rx = [1     0   0;
    0 cos(ypr(3)) -sin(ypr(3));
    0 sin(ypr(3)) cos(ypr(3))];

Rbe2 = Rz*Ry*Rx;
end

== matlab function quadcopter/Drone1/Subsystem/MATLAB Function2 ==
  data: R input; Jomega output; T input
function Jomega = Jmat(R, T)

Jomega = [R             zeros(3,3);
          zeros(3,3)        T];

end
